simulink model "OM2"  (R2019b)
settings: Solver=VariableStepAuto  StartTime=0.0  StopTime=t_final  MaxStep=0.001  RelTol=1e-3
values from neighbouring files (symbols this model uses):
  K1 = 1 + 0.1*(2*rand()-1)    [PI_regul.m]
  K2 = 1 + 0.1*(2*rand()-1)    [PI_regul.m]
  Kd = 1/(exp(T0/T2)-1)    [PI_regul.m]
  Ki = Kia*T0    [PI_regul.m]
  Kia = 1/(2*Tu*Kob)    [PI_regul.m]
  Kp = Kpa    [PI_regul.m]
  Kpa = T1/(2*Tu*Kob)    [PI_regul.m]
  st = 0    [PI_regul.m]
  T0 = 0.1    [PI_regul.m]
  T1 = 1 + 0.1*(2*rand()-1)    [PI_regul.m]
  T2 = 0.8 + 0.1*(2*rand()-1)    [PI_regul.m]
  Tur = T0/2    (= 0.05)    [PI_regul.m]
  Tzap = T0/2    (= 0.05)    [PI_regul.m]
settings Model: Creator=Anton Mayorov  LastModifiedBy=bedla
settings DataIOCC: ReturnWorkspaceOutputs=off
settings DebuggingCC: ArithmeticOperatorsInVariantConditions=warning
settings SFSimCC: SimUseLocalCustomCode=off  CustomCodeUndefinedFunction=UseInterfaceOnly
settings RTWCC: RTWUseLocalCustomCode=off

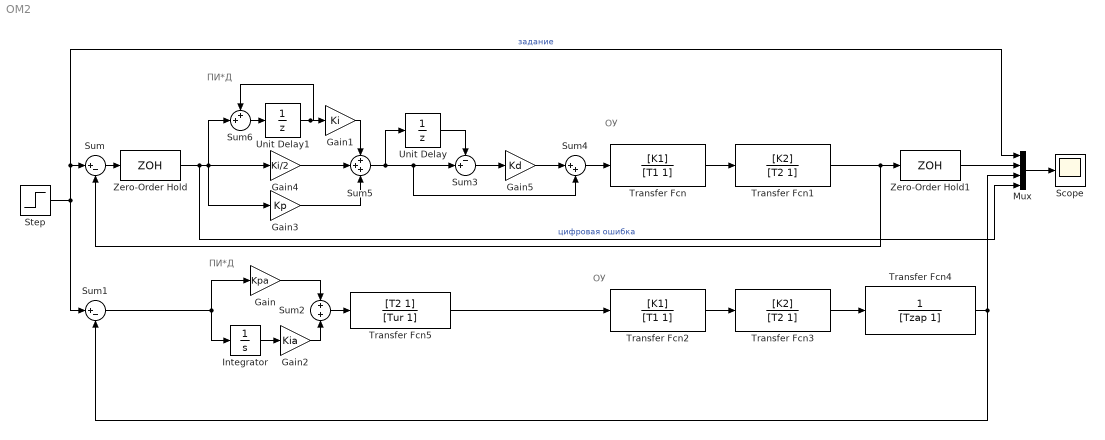
== system OM2 ==
  note: ОУ
  note: ОУ
  note: ПИ*Д
  note: ПИ*Д
  Gain : Gain  Gain=Kpa
  Gain1 : Gain  Gain=Ki
  Gain2 : Gain  Gain=Kia
  Gain3 : Gain  Gain=Kp
  Gain4 : Gain  Gain=Ki/2
  Gain5 : Gain  Gain=Kd
  Integrator : Integrator
  Mux : Mux
  Scope : Scope
  Step : Step  Time=st  SampleTime=0
  Sum : Sum  Inputs=|+-
  Sum1 : Sum  Inputs=|+-
  Sum2 : Sum
  Sum3 : Sum  Inputs=-+|
  Sum4 : Sum  Inputs=|++
  Sum5 : Sum  Inputs=+++
  Sum6 : Sum  Inputs=++|
  Transfer Fcn : TransferFcn  Numerator=[K1]  Denominator=[T1 1]
  Transfer Fcn1 : TransferFcn  Numerator=[K2]  Denominator=[T2 1]
  Transfer Fcn2 : TransferFcn  Numerator=[K1]  Denominator=[T1 1]
  Transfer Fcn3 : TransferFcn  Numerator=[K2]  Denominator=[T2 1]
  Transfer Fcn4 : TransferFcn  Denominator=[Tzap 1]
  Transfer Fcn5 : TransferFcn  Numerator=[T2 1]  Denominator=[Tur 1]
  Unit Delay : UnitDelay  SampleTime=T0  HasFrameUpgradeWarning=on
  Unit Delay1 : UnitDelay  SampleTime=-1  HasFrameUpgradeWarning=on
  Zero-Order Hold : ZeroOrderHold  SampleTime=T0
  Zero-Order Hold1 : ZeroOrderHold  SampleTime=T0
  wires:
  Zero-Order Hold/1 -> Gain4/1, Gain3/1, Sum6/2, Mux/4  "цифровая ошибка"
  Transfer Fcn/1 -> Transfer Fcn1/1
  Mux/1 -> Scope/1
  Transfer Fcn1/1 -> Sum/2, Zero-Order Hold1/1
  Sum/1 -> Zero-Order Hold/1
  Step/1 -> Mux/1, Sum/1, Sum1/1  "задание"
  Transfer Fcn3/1 -> Transfer Fcn4/1
  Transfer Fcn2/1 -> Transfer Fcn3/1
  Zero-Order Hold1/1 -> Mux/2
  Transfer Fcn4/1 -> Sum1/2, Mux/3
  Gain/1 -> Sum2/1
  Gain2/1 -> Sum2/2
  Sum1/1 -> Gain/1, Integrator/1
  Integrator/1 -> Gain2/1
  Sum2/1 -> Transfer Fcn5/1
  Transfer Fcn5/1 -> Transfer Fcn2/1
  Sum3/1 -> Gain5/1
  Sum4/1 -> Transfer Fcn/1
  Unit Delay/1 -> Sum3/1
  Gain1/1 -> Sum5/1
  Sum5/1 -> Sum4/2, Sum3/2, Unit Delay/1
  Gain5/1 -> Sum4/1
  Gain4/1 -> Sum5/2
  Gain3/1 -> Sum5/3
  Unit Delay1/1 -> Sum6/1, Gain1/1
  Sum6/1 -> Unit Delay1/1
